simulink model "mSimpleThermalStateSpace"  (R2021b)
settings: Solver=VariableStepAuto  StartTime=0.0  StopTime=10.0  RelTol=1e-3  AbsTol=1e-3
values from neighbouring files (symbols this model uses):
  CapMat = CaseData.CapMat    [tInterpolatedStateSpaceThermalModel.m]
  idx_TcoolantIn = 1    [tInterpolatedStateSpaceThermalModel.m]
  idx_TcoolantOut = 2    [tInterpolatedStateSpaceThermalModel.m]
  PowVec = [200;400;100]    [tInterpolatedStateSpaceThermalModel.m]
  ResMat = 1e9*ones(4,4)    [tCoolantHeatflowAdjustmentImplementation.m]    (also in tInterpolatedStateSpaceThermalModel.m = CaseData.ResMat)
  TcoolantIn = 300    [tInterpolatedStateSpaceThermalModel.m]
  TnodesInit = [TcoolantIn;330;290]    [tInterpolatedStateSpaceThermalModel.m]
libraries: fl_lib x11, ee_lib x3, nesl_utility x2, mcadROM_lib x1, simulink x1
settings Model: Creator=agonzale  LastModifiedBy=agonzale
settings SolverCC: AutoScaleAbsTol=off  AlgebraicLoopSolver=TrustRegion
settings DebuggingCC: SymbolicDimsDataTypeCodeGenerationDiagnostic=none  SFMachineParentedDataDiag=warning
settings SFSimCC: CustomCodeUndefinedFunction=UseInterfaceOnly
settings SimscapeCC: SimscapeLogType=all  SimscapeLogSimulationStatistics=on  SimscapeLogDataHistory=10000

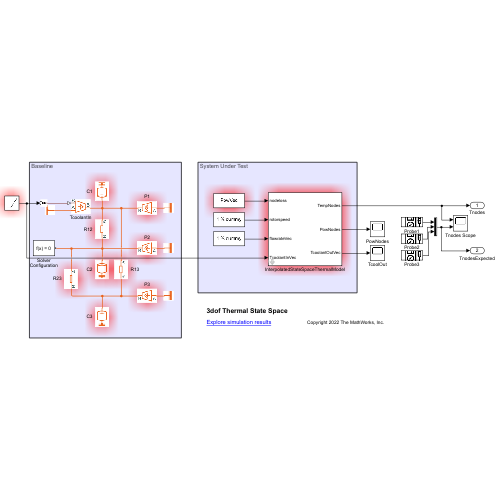
[thumbnail: Simulink's stored preview of the top-level diagram]
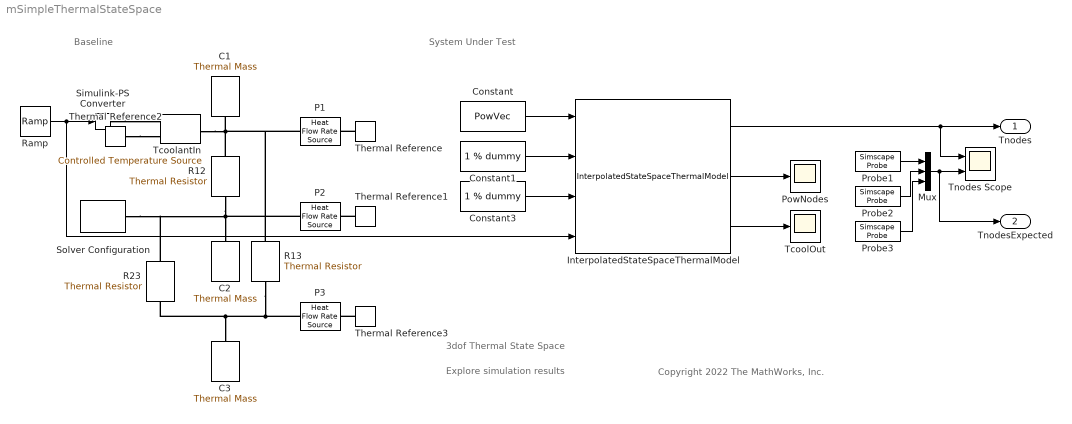
== system mSimpleThermalStateSpace ==
  note: System Under Test
  note: Baseline
  note: Explore simulation results
  note: 3dof Thermal State Space
  note: Copyright 2022 The MathWorks, Inc.
  C1 : fl_lib/Thermal/Thermal Elements/Thermal Mass  mass=CapMat(1) kg  sp_heat=1 J/(K*kg)  T_specify=on  T_priority=High  T=TnodesInit(1) K  T_nominal_specify=off  T_nominal_unit=K  T_nominal_value=1  Q_specify=off  Q_priority=None  Q=0 W  Q_nominal_specify=off  Q_nominal_unit=W  Q_nominal_value=1
  C2 : fl_lib/Thermal/Thermal Elements/Thermal Mass  mass=CapMat(2) kg  sp_heat=1 J/(K*kg)  T_specify=on  T_priority=High  T=TnodesInit(2) K  T_nominal_specify=off  T_nominal_unit=K  T_nominal_value=1  Q_specify=off  Q_priority=None  Q=0 W  Q_nominal_specify=off  Q_nominal_unit=W  Q_nominal_value=1
  C3 : fl_lib/Thermal/Thermal Elements/Thermal Mass  mass=CapMat(3) kg  sp_heat=1 J/(K*kg)  T_specify=on  T_priority=High  T=TnodesInit(3) K  T_nominal_specify=off  T_nominal_unit=K  T_nominal_value=1  Q_specify=off  Q_priority=None  Q=0 W  Q_nominal_specify=off  Q_nominal_unit=W  Q_nominal_value=1
  Constant : Constant  Value=PowVec
  Constant1 : Constant  Value=1 % dummy
  Constant3 : Constant  Value=1 % dummy
  InterpolatedStateSpaceThermalModel : mcadROM_lib/InterpolatedStateSpaceThermalModel  BkptsStruct=BkptsStruct  AMatND=AMatND  BMatND=BMatND  ResMatND=ResMatND  CoolAdjMat=AdjMat  CoolantArrayIdxs=[idx_TcoolantIn, idx_TcoolantOut]  InletCoolantIdxs=idx_TcoolantIn  OutletCoolantIdxs=idx_TcoolantOut  TnodesInit=TnodesInit
  Mux : Mux  Inputs=3
  P1 : fl_lib/Thermal/Thermal Sources/Heat Flow Rate Source  heat_flow=PowVec(1) W
      settings: SourceProductBaseCode=SS  InternalSimscapePortConfiguration="{\"Bottom\":[],\"Left\":[{\"id\":\"B\",\"label\":\"B\",\"type\":\"foundation.thermal.thermal\"}],\"Right\":[{\"id\":\"A\",\"label\":\"A\",\"type\":\"foundation.thermal.thermal\"}],\"Top\":[]}"
  P2 : fl_lib/Thermal/Thermal Sources/Heat Flow Rate Source  heat_flow=PowVec(2) W
      settings: SourceProductBaseCode=SS  InternalSimscapePortConfiguration="{\"Bottom\":[],\"Left\":[{\"id\":\"B\",\"label\":\"B\",\"type\":\"foundation.thermal.thermal\"}],\"Right\":[{\"id\":\"A\",\"label\":\"A\",\"type\":\"foundation.thermal.thermal\"}],\"Top\":[]}"
  P3 : fl_lib/Thermal/Thermal Sources/Heat Flow Rate Source  heat_flow=PowVec(3) W
      settings: SourceProductBaseCode=SS  InternalSimscapePortConfiguration="{\"Bottom\":[],\"Left\":[{\"id\":\"B\",\"label\":\"B\",\"type\":\"foundation.thermal.thermal\"}],\"Right\":[{\"id\":\"A\",\"label\":\"A\",\"type\":\"foundation.thermal.thermal\"}],\"Top\":[]}"
  PowNodes : Scope
  Probe1 : SimscapeProbe  BoundBlock=9  Variables={T}
  Probe2 : SimscapeProbe  BoundBlock=10  Variables={T}
  Probe3 : SimscapeProbe  BoundBlock=37  Variables={T}
  R12 : ee_lib/Passive/Thermal/Thermal Resistor  R=ResMat(1,2) K/W  T_specify=off  T_priority=None  T=0 K  T_nominal_specify=off  T_nominal_unit=K  T_nominal_value=1  Q_specify=off  Q_priority=None  Q=0 W  Q_nominal_specify=off  Q_nominal_unit=W  Q_nominal_value=1
      settings: SourceProductBaseCode=PS  InternalSimscapePortConfiguration="{\"Bottom\":[],\"Left\":[{\"id\":\"A\",\"label\":\"A\",\"type\":\"foundation.thermal.thermal\"}],\"Right\":[{\"id\":\"B\",\"label\":\"B\",\"type\":\"foundation.thermal.thermal\"}],\"Top\":[]}"
  R13 : ee_lib/Passive/Thermal/Thermal Resistor  R=ResMat(1,3) K/W  T_specify=off  T_priority=None  T=0 K  T_nominal_specify=off  T_nominal_unit=K  T_nominal_value=1  Q_specify=off  Q_priority=None  Q=0 W  Q_nominal_specify=off  Q_nominal_unit=W  Q_nominal_value=1
      settings: SourceProductBaseCode=PS  InternalSimscapePortConfiguration="{\"Bottom\":[],\"Left\":[{\"id\":\"A\",\"label\":\"A\",\"type\":\"foundation.thermal.thermal\"}],\"Right\":[{\"id\":\"B\",\"label\":\"B\",\"type\":\"foundation.thermal.thermal\"}],\"Top\":[]}"
  R23 : ee_lib/Passive/Thermal/Thermal Resistor  R=ResMat(2,3) K/W  T_specify=off  T_priority=None  T=0 K  T_nominal_specify=off  T_nominal_unit=K  T_nominal_value=1  Q_specify=off  Q_priority=None  Q=0 W  Q_nominal_specify=off  Q_nominal_unit=W  Q_nominal_value=1
      settings: SourceProductBaseCode=PS  InternalSimscapePortConfiguration="{\"Bottom\":[],\"Left\":[{\"id\":\"A\",\"label\":\"A\",\"type\":\"foundation.thermal.thermal\"}],\"Right\":[{\"id\":\"B\",\"label\":\"B\",\"type\":\"foundation.thermal.thermal\"}],\"Top\":[]}"
  Ramp : simulink/Sources/Ramp  slope=10  start=5  InitialOutput=TcoolantIn
  Simulink-PS Converter : nesl_utility/Simulink-PS Converter  PhysicalDomain=network_engine_domain  SubClassName=ps_input  LeftPortType=input  RightPortType=output  PseudoPeriodic=off  Frequencies=[]  NoiseDistribution=none  NoiseParameters=[]  Unit=K  AffineConversion=off  FilteringAndDerivatives=filter  SimscapeFilterOrder=1  InputFilterTimeConstant=1e-4  UdotUserProvided=0
      settings: SourceProductBaseCode=PW,SS
  Solver Configuration : nesl_utility/Solver Configuration  PhysicalDomain=network_engine_domain  SubClassName=solver  LeftPortType=input  RightPortType=generic  Tones=[]  Harmonics=[]  SimulateNoise=off  Profile=off  UseLocalSampling=off  EnableSwitchedLinearOptims=on  FrequencyDomain=off  UseCCode=off  RelTol=0.001  AbsTol=1e-06  MinStep=1e-09  ToWorkspace=off  RevertToSquareIcSolve=off  NumHomotopyIterations=100  PhasorMode=off  PhasorModeNumHarmonics=1  DoDC=off  ResidualTolerance=1e-09  UseLocalSolver=off  LocalSolverChoice=NE_BACKWARD_EULER_ADVANCER  LocalSolverSampleTime=0.001  DoFixedCost=off  MaxNonlinIter=3  MaxModeIter=2  ComputeImpulses=off  ImpulseIterations=2  LinearAlgebra=auto  EquationFormulation=NE_TIME_EF  DelaysMemoryBudget=1024  AutomaticFiltering=on  FilteringTimeConstant=0.001  PartitionStorageMethod=AS_NEEDED  PartitionMemoryBudget=1024  PartitionMethod=ROBUST
      settings: SourceProductBaseCode=PW,SS
  TcoolOut : Scope
  TcoolantIn : fl_lib/Thermal/Thermal Sources/Controlled Temperature Source
  Thermal Reference{,1..3} (4 alike) : fl_lib/Thermal/Thermal Elements/Thermal Reference
  Tnodes Scope : Scope  NumInputPorts=2
  Tnodes : Outport
  TnodesExpected : Outport  Port=2
  wires:
  Constant/1 -> InterpolatedStateSpaceThermalModel/1
  Constant1/1 -> InterpolatedStateSpaceThermalModel/2
  Ramp/1 -> Simulink-PS Converter/1, InterpolatedStateSpaceThermalModel/4
  InterpolatedStateSpaceThermalModel/1 -> Tnodes Scope/1, Tnodes/1
  Mux/1 -> TnodesExpected/1, Tnodes Scope/2
  Probe1/1 -> Mux/1
  Probe2/1 -> Mux/2
  Probe3/1 -> Mux/3
  InterpolatedStateSpaceThermalModel/3 -> TcoolOut/1
  Constant3/1 -> InterpolatedStateSpaceThermalModel/3
  InterpolatedStateSpaceThermalModel/2 -> PowNodes/1
  connections:
  R12/LConn1 -- P1/LConn1 -- R13/LConn1 -- TcoolantIn/LConn1 -- C1/LConn1
  R12/RConn1 -- Solver Configuration/RConn1 -- R23/LConn1 -- C2/LConn1 -- P2/LConn1
  Thermal Reference/LConn1 -- P1/RConn1
  Thermal Reference1/LConn1 -- P2/RConn1
  Simulink-PS Converter/RConn1 -- TcoolantIn/RConn1
  Thermal Reference2/LConn1 -- TcoolantIn/RConn2
  P3/LConn1 -- R13/RConn1 -- R23/RConn1 -- C3/LConn1
  Thermal Reference3/LConn1 -- P3/RConn1
